simulink model "pend_HINF_JW"  (R2018b)
settings: Solver=FixedStepAuto  StartTime=0.0  StopTime=T_final  FixedStep=h  RelTol=1e-3  EnableMultiTasking=on
PreLoadFcn:
  | hwinit
StartFcn:
  | hwinit
values from neighbouring files (symbols this model uses):
  adingain = [1 1]    [HINF_Changing_ref_2.mat]    (also in HINF_Constant_ref_3.mat)
  adinoffs = [-0.2676 -0.1614]    [HINF_Changing_ref_2.mat]    (also in HINF_Constant_ref_3.mat)
  angle_bound = [0.287979326579 0 -0.226892802759]    [HINF_Changing_ref_2.mat]    (also in HINF_Constant_ref_3.mat)
  angle_real = [-0.0759 0.0004 0.064]    [HINF_Changing_ref_2.mat]    (also in HINF_Constant_ref_3.mat)
  d_cart = 6.04305713102    [HINF_Changing_ref_2.mat]    (also in HINF_Constant_ref_3.mat)
  d_pend = 0.0423602307049    [HINF_Changing_ref_2.mat]    (also in HINF_Constant_ref_3.mat)
  daoutgain = 0.9    [HINF_Changing_ref_2.mat]    (also in HINF_Constant_ref_3.mat)
  daoutoffs = 0    [HINF_Changing_ref_2.mat]    (also in HINF_Constant_ref_3.mat)
  h = 0.001    [HINF_Changing_ref_2.mat]    (also in HINF_Constant_ref_3.mat)
  Km = 5.94193675955    [HINF_Changing_ref_2.mat]    (also in HINF_Constant_ref_3.mat)
  l = 0.6    [HINF_Changing_ref_2.mat]    (also in HINF_Constant_ref_3.mat)
  mc = 0.664927729397    [HINF_Changing_ref_2.mat]    (also in HINF_Constant_ref_3.mat)
  mp = 0.175046141792    [HINF_Changing_ref_2.mat]    (also in HINF_Constant_ref_3.mat)
  option = 1    [HINF_Changing_ref_2.mat]    (also in HINF_Constant_ref_3.mat; main_Hinf.m; main_Hinf_JW.m; main_Hinf_JW2.m)
  pend = [-0.573 -0.559 -0.487 -0.418 -0.353 -0.29 -0.225 -0.16 -0.094 -0.0247 -0.0037]    [HINF_Changing_ref_2.mat]    (also in HINF_Constant_ref_3.mat)
  T_final = 40    [HINF_Changing_ref_2.mat]    (also in HINF_Constant_ref_3.mat; main_Hinf.m; main_Hinf_JW.m; main_Hinf_JW2.m)
  x_init = [0.601318509615 0 0.00620401072168 0]    [HINF_Changing_ref_2.mat]    (also in HINF_Constant_ref_3.mat = [0.497578125 0 -0.00458757804321 0]; main_Hinf.m = [Pos_Pendulum.data(1),0,Angle_Pendulum.data(1),0]; main_Hinf_JW.m = [Pos_Pendulum.data(1),0,Angle_Pendulum.data(1),0]; main_Hinf_JW2.m = [Pos_Pendulum.data(1),0,Angle_Pendulum.data(1),0])
undefined symbols (not defined in the file or in its folder): Advantech, PCI
libraries: sldrtlib x2, cstblocks x1
settings Model: Creator=zhidayat  LastModifiedBy=mdepont
settings DataIOCC: LimitDataPoints=on  SaveFormat=Array
settings OptimizationCC: ExpressionDepthLimit=2147483647  LifeSpan=inf
settings DebuggingCC: AllowSymbolicDim=off  StateNameClashWarn=warning  StrictBusMsg=ErrorOnBusTreatedAsVector  SFUnexpectedBacktrackingDiag=warning  SFNoUnconditionalDefaultTransitionDiag=warning  SFExecutionAtInitializationDiag=none
settings HardwareCC: ProdBitPerPointer=32  ProdBitPerSizeT=32  ProdBitPerPtrDiffT=32  ProdLargestAtomicFloat=None  ProdIntDivRoundTo=Undefined  ProdEndianess=Unspecified  ProdWordSize=32  ProdHWDeviceType=32-bit Generic
settings ModelReferenceCC: PropagateSignalLabelsOutOfModel=off
settings SFSimCC: SimUseLocalCustomCode=off
settings RTWCC: RTWUseLocalCustomCode=off
settings CodeAppCC: StateflowObjectComments=on
settings GRTTargetCC: TargetLangStandard=C89/C90 (ANSI)  GeneratePreprocessorConditionals=Disable all  CombineOutputUpdateFcns=off  GRTInterface=on
settings ConfigComp: CovMetricSettings=dw  CovHtmlReporting=on  CovSaveCumulativeToWorkspaceVar=on  CovSaveSingleToWorkspaceVar=on  CovExternalEMLEnable=off

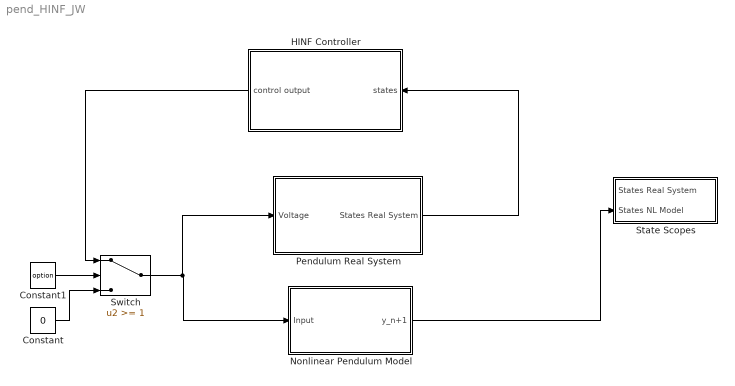
== system pend_HINF_JW ==
  Constant : Constant  Value=0
  Constant1 : Constant  Value=option
  HINF Controller : Subsystem
  Nonlinear Pendulum Model : Subsystem
  "Pendulum Real System " : Subsystem
  "State Scopes " : Subsystem
  Switch : Switch  Threshold=1
  wires:
  Nonlinear Pendulum Model/1(y_n+1) -> "State Scopes "/2(States NL Model)
  Constant/1 -> Switch/3
  Constant1/1 -> Switch/2
  HINF Controller/1("control output ") -> Switch/1
  Switch/1 -> Nonlinear Pendulum Model/1(Input), "Pendulum Real System "/1(Voltage)
  "Pendulum Real System "/1(States Real System) -> HINF Controller/1(states)

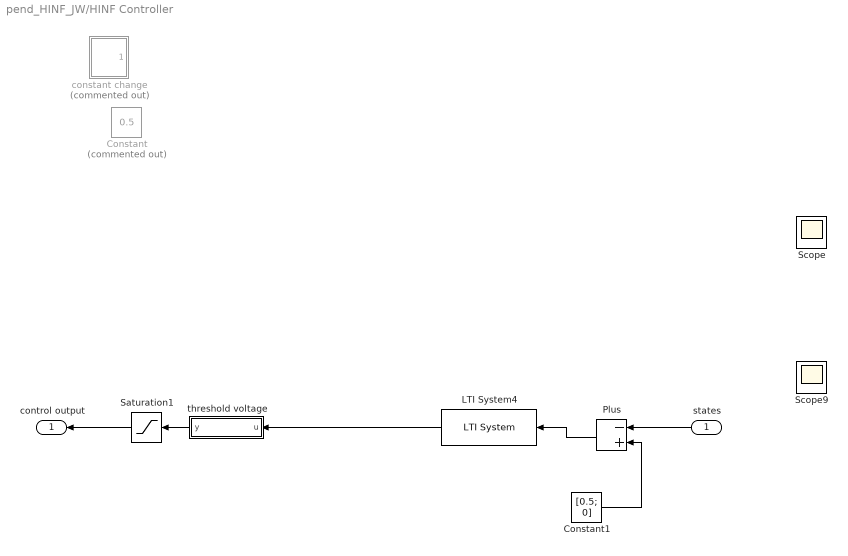
== system pend_HINF_JW/HINF Controller ==
  states : Inport
  Constant : Constant  Commented=on  Value=0.5
  Constant1 : Constant  Value=[0.5; 0]
  LTI System4 : cstblocks/LTI System  sys=K_d  IC=[]
  Plus : Sum  Inputs=-+
  Saturation1 : Saturate  UpperLimit=1  LowerLimit=-1
  Scope : Scope
  Scope9 : Scope
  "constant change " : Subsystem  Commented=on
  threshold voltage : MATLAB Function  TreatAsAtomicUnit=on
  "control output " : Outport
  wires:
  Saturation1/1 -> "control output "/1
  ? -> Scope/1
  ? -> Scope9/1
  LTI System4/1 -> threshold voltage/1(u)
  threshold voltage/1(y) -> Saturation1/1
  states/1 -> Plus/1
  Plus/1 -> LTI System4/1
  Constant1/1 -> Plus/2

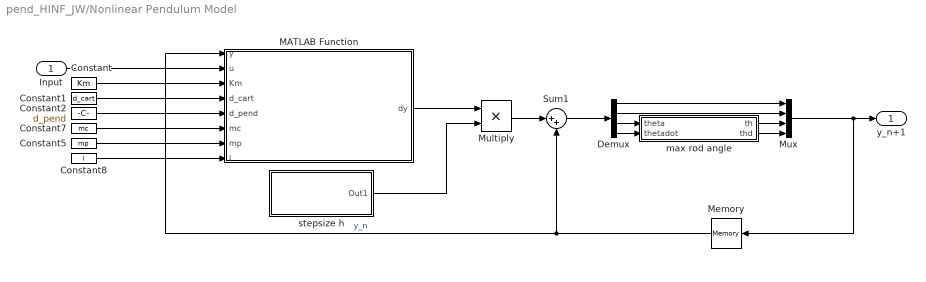
== system pend_HINF_JW/Nonlinear Pendulum Model ==
  Input : Inport
  Constant : Constant  Value=Km
  Constant1 : Constant  Value=d_cart
  Constant2 : Constant  Value=d_pend
  Constant5 : Constant  Value=mp
  Constant7 : Constant  Value=mc
  Constant8 : Constant  Value=l  SampleTime=h
  Demux : Demux
  MATLAB Function : MATLAB Function  TreatAsAtomicUnit=on
  Memory : Memory  InitialCondition=x_init
  Multiply : Product
  Mux : Mux
  Sum1 : Sum  Inputs=|++
  max rod angle : MATLAB Function  TreatAsAtomicUnit=on
  stepsize h : Subsystem
  y_n+1 : Outport
  wires:
  Multiply/1 -> Sum1/1
  Memory/1 -> MATLAB Function/1(y), Sum1/2  "y_n"
  stepsize h/1(Out1) -> Multiply/2
  Constant/1 -> MATLAB Function/3(Km)
  Constant1/1 -> MATLAB Function/4(d_cart)
  Sum1/1 -> Demux/1
  Demux/2 -> Mux/2
  Demux/1 -> Mux/1
  Input/1 -> MATLAB Function/2(u)
  Constant2/1 -> MATLAB Function/5(d_pend)
  MATLAB Function/1(dy) -> Multiply/1
  Constant5/1 -> MATLAB Function/7(mp)
  Constant7/1 -> MATLAB Function/6(mc)
  Constant8/1 -> MATLAB Function/8(l)
  Demux/3 -> max rod angle/1(theta)
  Demux/4 -> max rod angle/2(thetadot)
  Mux/1 -> y_n+1/1, Memory/1
  max rod angle/1(th) -> Mux/3
  max rod angle/2(thd) -> Mux/4

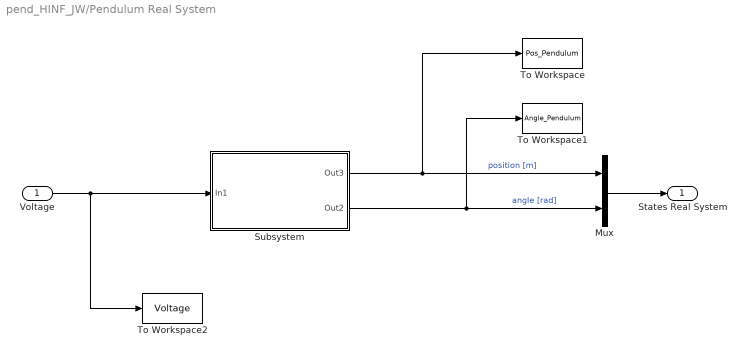
== system pend_HINF_JW/Pendulum Real System  ==
  Voltage : Inport
  Mux : Mux  Inputs=2
  Subsystem : Subsystem  InitFcn=hwinit  StartFcn=hwinit  mask{h=h}
      mask prompts: h "Sample time"
      mask init:
      | hwinit
      mask Display: disp('Pendulum');
  To Workspace : ToWorkspace  VariableName=Pos_Pendulum  SaveFormat=Timeseries  SampleTime=-1
  To Workspace1 : ToWorkspace  VariableName=Angle_Pendulum  SaveFormat=Timeseries  SampleTime=-1
  To Workspace2 : ToWorkspace  VariableName=Voltage  SaveFormat=Timeseries  SampleTime=-1
  States Real System : Outport
  wires:
  Voltage/1 -> To Workspace2/1, Subsystem/1(In1)
  Subsystem/1(Out3) -> To Workspace/1, Mux/1  "position [m]"
  Subsystem/2(Out2) -> Mux/2, To Workspace1/1  "angle [rad]"
  Mux/1 -> States Real System/1

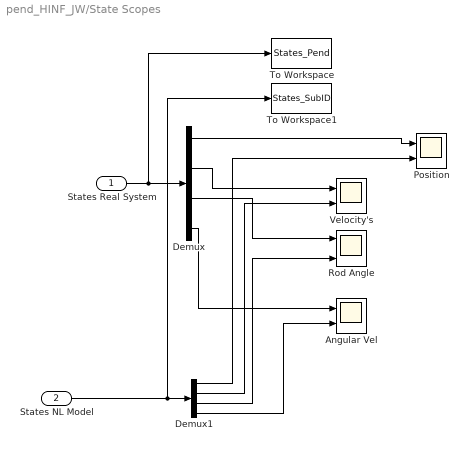
== system pend_HINF_JW/State Scopes  ==
  States Real System : Inport
  States NL Model : Inport  Port=2
  "Angular Vel " : Scope  NumInputPorts=2
  Demux : Demux
  Demux1 : Demux
  Position : Scope  NumInputPorts=2
  Rod Angle : Scope  NumInputPorts=2
  To Workspace : ToWorkspace  VariableName=States_Pend  SaveFormat=Timeseries  SampleTime=-1
  To Workspace1 : ToWorkspace  VariableName=States_SubID  SaveFormat=Timeseries  SampleTime=h
  Velocity's : Scope  NumInputPorts=2
  wires:
  States Real System/1 -> To Workspace/1, Demux/1
  Demux/1 -> Position/1
  States NL Model/1 -> To Workspace1/1, Demux1/1
  Demux1/2 -> Velocity's/2
  Demux/2 -> Velocity's/1
  Demux/3 -> Rod Angle/1
  Demux1/3 -> Rod Angle/2
  Demux/4 -> "Angular Vel "/1
  Demux1/4 -> "Angular Vel "/2
  Demux1/1 -> Position/2

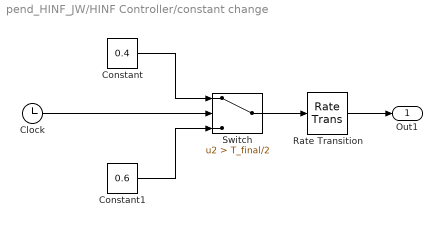
== system pend_HINF_JW/HINF Controller/constant change  ==
  Clock : Clock
  Constant : Constant  Value=0.4
  Constant1 : Constant  Value=0.6
  Rate Transition : RateTransition  OutPortSampleTime=h
  Switch : Switch  Criteria=u2 > Threshold  Threshold=T_final/2
  Out1 : Outport
  wires:
  Constant/1 -> Switch/1
  Constant1/1 -> Switch/3
  Clock/1 -> Switch/2
  Switch/1 -> Rate Transition/1
  Rate Transition/1 -> Out1/1

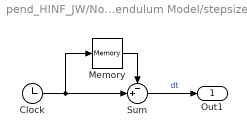
== system pend_HINF_JW/Nonlinear Pendulum Model/stepsize h ==
  Clock : Clock
  Memory : Memory
  Sum : Sum  Inputs=-+|
  Out1 : Outport
  wires:
  Memory/1 -> Sum/1
  Sum/1 -> Out1/1  "dt"
  Clock/1 -> Memory/1, Sum/2

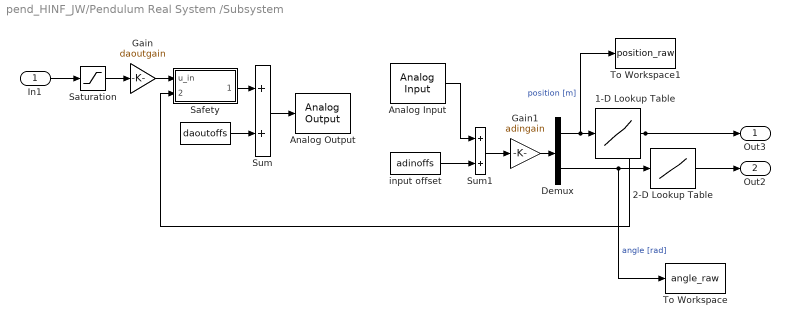
== system pend_HINF_JW/Pendulum Real System /Subsystem ==
  In1 : Inport
  " " : Constant  Value=daoutoffs
  1-D Lookup Table : Lookup_n-D  NumberOfTableDimensions=1  BreakpointsForDimension1=pend  Table=real  InternalRulePriority=Speed  RndMeth=Simplest  InputSameDT=on
  2-D Lookup Table : Lookup_n-D  NumberOfTableDimensions=1  BreakpointsForDimension1=angle_real  BreakpointsForDimension2=[1:3]  Table=angle_bound  InternalRulePriority=Speed  RndMeth=Simplest  InputSameDT=on
  Analog Input : sldrtlib/Analog Input  SampleTime=h  MaxMissedTicks=ticklost  ShowMissedTicks=off  YieldWhenWaiting=on  DrvName=Advantech/PCI-1711  DrvAddress=4294967295  DrvOptions=zeros(1,0)  Channels=adinchannels  RangeMode=2  VoltRange=1  DataType=1
      settings: AttributesFormatString=Advantech\nPCI-1711 [auto]  SourceProductName=Simulink Desktop Real-Time
  Analog Output : sldrtlib/Analog Output  SampleTime=h  MaxMissedTicks=ticklost  ShowMissedTicks=off  YieldWhenWaiting=off  DrvName=Advantech/PCI-1711  DrvAddress=4294967295  DrvOptions=zeros(1,0)  Channels=daoutchannels  RangeMode=2  VoltRange=2  InitialValue=0  FinalValue=0
      settings: AttributesFormatString=Advantech\nPCI-1711 [auto]  SourceProductName=Simulink Desktop Real-Time
  Demux : Demux  Outputs=2
  Gain : Gain  Gain=daoutgain  SaturateOnIntegerOverflow=on  OutDataTypeStr=Inherit: Same as input  ParamDataTypeStr=Inherit: Same as input
  Gain1 : Gain  Gain=adingain  SaturateOnIntegerOverflow=on  OutDataTypeStr=Inherit: Same as input  ParamDataTypeStr=Inherit: Same as input
  Safety : Subsystem
      mask help: The output of the block is restricted to prevent damage to the system. If the cart reaches some safety margins (left: -0.26 and right: 0.26), the output of the block is nullifed. Then the control has to be restarted.
      mask Display: disp('Safety \n margins')
  Saturation : Saturate  UpperLimit=1  LowerLimit=-1
  Sum : Sum  SaturateOnIntegerOverflow=on  OutDataTypeStr=Inherit: Same as first input
  Sum1 : Sum  SaturateOnIntegerOverflow=on  InputSameDT=on  OutDataTypeStr=Inherit: Same as first input
  To Workspace : ToWorkspace  VariableName=angle_raw  SaveFormat=Timeseries  SampleTime=-1
  To Workspace1 : ToWorkspace  VariableName=position_raw  SaveFormat=Timeseries  SampleTime=-1
  input offset : Constant  Value=adinoffs
  Out3 : Outport
  Out2 : Outport  Port=2
  wires:
  Sum1/1 -> Gain1/1
  input offset/1 -> Sum1/2
  Analog Input/1 -> Sum1/1
  Gain1/1 -> Demux/1
  Saturation/1 -> Gain/1
  Sum/1 -> Analog Output/1
  " "/1 -> Sum/2
  In1/1 -> Saturation/1
  Demux/2 -> 2-D Lookup Table/1, To Workspace/1  "angle [rad]"
  Safety/1(u_out) -> Sum/1
  Gain/1 -> Safety/1(u_in)
  Demux/1 -> To Workspace1/1, 1-D Lookup Table/1  "position [m]"
  1-D Lookup Table/1 -> Safety/2(Position), Out3/1
  2-D Lookup Table/1 -> Out2/1

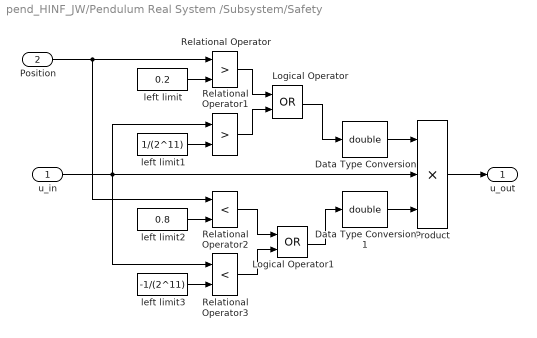
== system pend_HINF_JW/Pendulum Real System /Subsystem/Safety ==
  u_in : Inport
  Position : Inport  Port=2
  Data Type Conversion : DataTypeConversion  OutDataTypeStr=double
  Data Type Conversion1 : DataTypeConversion  OutDataTypeStr=double
  Logical Operator : Logic  Operator=OR  OutDataTypeStr=boolean
  Logical Operator1 : Logic  Operator=OR  OutDataTypeStr=boolean
  Product : Product  Inputs=3  SaturateOnIntegerOverflow=on  InputSameDT=on  OutDataTypeStr=Inherit: Same as first input
  Relational Operator : RelationalOperator  Operator=>  OutDataTypeStr=boolean  RndMeth=Nearest  InputSameDT=on
  Relational Operator1 : RelationalOperator  Operator=>  OutDataTypeStr=boolean  RndMeth=Nearest  InputSameDT=on
  Relational Operator2 : RelationalOperator  Operator=<  OutDataTypeStr=boolean  RndMeth=Nearest  InputSameDT=on
  Relational Operator3 : RelationalOperator  Operator=<  OutDataTypeStr=boolean  RndMeth=Nearest  InputSameDT=on
  left limit : Constant  Value=0.2
  left limit1 : Constant  Value=1/(2^11)
  left limit2 : Constant  Value=0.8
  left limit3 : Constant  Value=-1/(2^11)
  u_out : Outport
  wires:
  left limit1/1 -> Relational Operator1/2
  u_in/1 -> Relational Operator1/1, Relational Operator3/1, Product/2
  Logical Operator1/1 -> Data Type Conversion1/1
  Logical Operator/1 -> Data Type Conversion/1
  left limit/1 -> Relational Operator/2
  Relational Operator/1 -> Logical Operator/1
  Relational Operator1/1 -> Logical Operator/2
  Position/1 -> Relational Operator/1, Relational Operator2/1
  left limit2/1 -> Relational Operator2/2
  Relational Operator2/1 -> Logical Operator1/1
  left limit3/1 -> Relational Operator3/2
  Relational Operator3/1 -> Logical Operator1/2
  Product/1 -> u_out/1
  Data Type Conversion/1 -> Product/1
  Data Type Conversion1/1 -> Product/3

== matlab function pend_HINF_JW/Nonlinear Pendulum Model/MATLAB Function ==
  data: y input; u input; dy output; Km input; d_cart input; d_pend input; mc input; mp input; l input
function dy = nl_pend_dynamics(y,u,Km,d_cart,d_pend,mc,mp,l)
g = 9.81;
dy = zeros(4,1);

dy(1,1) = y(2);
dy(2,1) = 1/((mc+mp)*(1-0.75*mp))*(Km*u - d_cart*y(2) + 3/(2*l)*((l/2)*mp*g*y(3) - d_pend*y(4)) + mp*l*y(4)^2*y(3)/2);
dy(3,1) = y(4);
dy(4,1) = 3/(mp*l^2)*(l*mp*dy(2,1)/2 + l*mp*g*y(3)/2 - d_pend*y(4));

== matlab function pend_HINF_JW/HINF Controller/threshold voltage ==
  data: u input; y output
function y = fcn(u)
ub_mtr_threshold = 0.26;
       y = u + sign(u)*0.1*ub_mtr_threshold;
%        if abs(u) <= ub_mtr_threshold && abs(u) >= lb_mtr_threshold
%            y = sign(u)*(ub_mtr_threshold + 0.02);
%        elseif abs(u) <= lb_mtr_threshold
%            y = 0;
%        else 
%            y = u;
%        end
end

== matlab function pend_HINF_JW/Nonlinear Pendulum Model/max rod angle ==
  data: theta input; th output; thetadot input; thd output
function [th,thd] = fcn(theta, thetadot)
threshold = 0.26;

if abs(theta) > threshold
    th = threshold*sign(theta);
    thd = 0;
else
    th = theta;
    thd = thetadot;
end
